simulink model "sm_DynamicCompression"  (R2019b)
settings: Solver=FixedStepDiscrete  StartTime=0.0  StopTime=stop_time  RelTol=1e-3
InitFcn:
  | sm_callback_init
StopFcn:
  | sm_callback_stop
values from neighbouring files (symbols this model uses):
  a = 100*(r^2)    [InitializeCompressionSettings.m]    (also in sm_check_control_signals.m = registers(i).(supplied_fields{j}); sm_check_control_signals_LOCAL_1434.m = registers(i).(supplied_fields{j}))
  B_k_0_init = zeros(1,FIR_0_Uprate)    [sm_callback_init.m]
  B_k_1_init = zeros(1,FIR_0_Uprate)    [sm_callback_init.m]
  B_k_2_init = zeros(1,FIR_0_Uprate)    [sm_callback_init.m]
  B_k_3_init = zeros(1,FIR_0_Uprate)    [sm_callback_init.m]
  B_k_4_init = zeros(1,FIR_0_Uprate)    [sm_callback_init.m]
  B_k_5_init = zeros(1,FIR_0_Uprate)    [sm_callback_init.m]
  calib_bpfs = bpfs    [sm_compression_init.m]
  delayFix = maxDelay-delays    [Initialize_Delay_Values.m]
  F_bits = 28    [TestingLibraryScripts.m]    (also in sm_compression_init.m)
  FIR_0_Size = (ceil(log2(length(calib_bpfs(2:calib_bpfs(1,1)+1 ,1)'))))    [sm_callback_init.m]
  FIR_0_Uprate = 2^FIR_0_Size    [sm_callback_init.m]
  M_bits = 1    [TestingLibraryScripts.m]    (also in sm_compression_init.m = 5)
  M_Bits = M_bits    (= 5)    [sm_compression_init.m]
  mp = sm_init_avalon_signals(mp)    [sm_callback_init.m]
  r_att = nthroot(0.1, s_att)    [sm_compression_init.m]
  r_rel = nthroot(0.1, s_rel)    [sm_compression_init.m]
  recombGain = ones(1,NChans)    [sm_compression_init.m]
  TABLE_SEL_BYPASS_ENABLE = 0    [sm_callback_init.m]
  Ts = mp.Ts    [sm_compression_init.m]
  Ts_system = mp.Ts_system    [sm_compression_init.m]
  W_bits = 32    [TestingLibraryScripts.m]    (also in sm_compression_init.m)
  X_high = 1    [sm_compression_init.m]
undefined symbols (not defined in the file or in its folder): b, c, Gain_Table, ig_eq
libraries: hdlsllib x272, simulink x127, dsphdlfiltering x2
(part 6 of 8)

== system sm_DynamicCompression/dataplane/Avalon Data Processing/Left Channel Processing/recalculate/Nchan_FbankAGC_AID/Compression_4/Compression_Gain_Calc/Linear_Approximation/LSR(N) ==
  NShifts : Inport
  x_in : Inport  Port=2
  Bit Rotate : hdlsllib/Logic and Bit Operations/Bit Rotate  mode=Rotate Right  N=1
      settings: SourceProductName=Simulink  SourceProductBaseCode=SL
  Bit Rotate1 : hdlsllib/Logic and Bit Operations/Bit Rotate  mode=Rotate Right  N=2
      settings: SourceProductName=Simulink  SourceProductBaseCode=SL
  Bit Rotate10 : hdlsllib/Logic and Bit Operations/Bit Rotate  mode=Rotate Right  N=11
      settings: SourceProductName=Simulink  SourceProductBaseCode=SL
  Bit Rotate11 : hdlsllib/Logic and Bit Operations/Bit Rotate  mode=Rotate Right  N=12
      settings: SourceProductName=Simulink  SourceProductBaseCode=SL
  Bit Rotate12 : hdlsllib/Logic and Bit Operations/Bit Rotate  mode=Rotate Right  N=13
      settings: SourceProductName=Simulink  SourceProductBaseCode=SL
  Bit Rotate13 : hdlsllib/Logic and Bit Operations/Bit Rotate  mode=Rotate Right  N=14
      settings: SourceProductName=Simulink  SourceProductBaseCode=SL
  Bit Rotate14 : hdlsllib/Logic and Bit Operations/Bit Rotate  mode=Rotate Right  N=15
      settings: SourceProductName=Simulink  SourceProductBaseCode=SL
  Bit Rotate2 : hdlsllib/Logic and Bit Operations/Bit Rotate  mode=Rotate Right  N=3
      settings: SourceProductName=Simulink  SourceProductBaseCode=SL
  Bit Rotate3 : hdlsllib/Logic and Bit Operations/Bit Rotate  mode=Rotate Right  N=4
      settings: SourceProductName=Simulink  SourceProductBaseCode=SL
  Bit Rotate4 : hdlsllib/Logic and Bit Operations/Bit Rotate  mode=Rotate Right  N=5
      settings: SourceProductName=Simulink  SourceProductBaseCode=SL
  Bit Rotate5 : hdlsllib/Logic and Bit Operations/Bit Rotate  mode=Rotate Right  N=6
      settings: SourceProductName=Simulink  SourceProductBaseCode=SL
  Bit Rotate6 : hdlsllib/Logic and Bit Operations/Bit Rotate  mode=Rotate Right  N=7
      settings: SourceProductName=Simulink  SourceProductBaseCode=SL
  Bit Rotate7 : hdlsllib/Logic and Bit Operations/Bit Rotate  mode=Rotate Right  N=8
      settings: SourceProductName=Simulink  SourceProductBaseCode=SL
  Bit Rotate8 : hdlsllib/Logic and Bit Operations/Bit Rotate  mode=Rotate Right  N=9
      settings: SourceProductName=Simulink  SourceProductBaseCode=SL
  Bit Rotate9 : hdlsllib/Logic and Bit Operations/Bit Rotate  mode=Rotate Right  N=10
      settings: SourceProductName=Simulink  SourceProductBaseCode=SL
  Multiport Switch : MultiPortSwitch  DataPortOrder=Zero-based contiguous  Inputs=16  DiagnosticForDefault=Warning  zeroidx=on
  x_shifted : Outport  VectorParamsAs1DForOutWhenUnconnected=off
  wires:
  NShifts/1 -> Multiport Switch/1
  Multiport Switch/1 -> x_shifted/1
  x_in/1 -> Bit Rotate12/1, Bit Rotate13/1, Bit Rotate14/1, Bit Rotate11/1, Bit Rotate10/1, Bit Rotate9/1, Bit Rotate8/1, Bit Rotate7/1, Bit Rotate5/1, Bit Rotate4/1, Multiport Switch/2, Bit Rotate/1, Bit Rotate1/1, Bit Rotate2/1, Bit Rotate3/1, Bit Rotate6/1
  Bit Rotate/1 -> Multiport Switch/3
  Bit Rotate1/1 -> Multiport Switch/4
  Bit Rotate2/1 -> Multiport Switch/5
  Bit Rotate3/1 -> Multiport Switch/6
  Bit Rotate4/1 -> Multiport Switch/7
  Bit Rotate5/1 -> Multiport Switch/8
  Bit Rotate6/1 -> Multiport Switch/9
  Bit Rotate7/1 -> Multiport Switch/10
  Bit Rotate8/1 -> Multiport Switch/11
  Bit Rotate9/1 -> Multiport Switch/12
  Bit Rotate10/1 -> Multiport Switch/13
  Bit Rotate11/1 -> Multiport Switch/14
  Bit Rotate12/1 -> Multiport Switch/15
  Bit Rotate13/1 -> Multiport Switch/16
  Bit Rotate14/1 -> Multiport Switch/17

== system sm_DynamicCompression/dataplane/Avalon Data Processing/Left Channel Processing/recalculate/Nchan_FbankAGC_AID/Compression_4/Compression_Gain_Calc/LogAddressing/LSL(N) ==
  NShifts : Inport
  x_in : Inport  Port=2
  Bit Rotate : hdlsllib/Logic and Bit Operations/Bit Rotate  mode=Rotate Left  N=1
      settings: SourceProductName=Simulink  SourceProductBaseCode=SL
  Bit Rotate1 : hdlsllib/Logic and Bit Operations/Bit Rotate  mode=Rotate Left  N=2
      settings: SourceProductName=Simulink  SourceProductBaseCode=SL
  Bit Rotate10 : hdlsllib/Logic and Bit Operations/Bit Rotate  mode=Rotate Left  N=11
      settings: SourceProductName=Simulink  SourceProductBaseCode=SL
  Bit Rotate11 : hdlsllib/Logic and Bit Operations/Bit Rotate  mode=Rotate Left  N=12
      settings: SourceProductName=Simulink  SourceProductBaseCode=SL
  Bit Rotate12 : hdlsllib/Logic and Bit Operations/Bit Rotate  mode=Rotate Left  N=13
      settings: SourceProductName=Simulink  SourceProductBaseCode=SL
  Bit Rotate13 : hdlsllib/Logic and Bit Operations/Bit Rotate  mode=Rotate Left  N=14
      settings: SourceProductName=Simulink  SourceProductBaseCode=SL
  Bit Rotate14 : hdlsllib/Logic and Bit Operations/Bit Rotate  mode=Rotate Left  N=15
      settings: SourceProductName=Simulink  SourceProductBaseCode=SL
  Bit Rotate2 : hdlsllib/Logic and Bit Operations/Bit Rotate  mode=Rotate Left  N=3
      settings: SourceProductName=Simulink  SourceProductBaseCode=SL
  Bit Rotate3 : hdlsllib/Logic and Bit Operations/Bit Rotate  mode=Rotate Left  N=4
      settings: SourceProductName=Simulink  SourceProductBaseCode=SL
  Bit Rotate4 : hdlsllib/Logic and Bit Operations/Bit Rotate  mode=Rotate Left  N=5
      settings: SourceProductName=Simulink  SourceProductBaseCode=SL
  Bit Rotate5 : hdlsllib/Logic and Bit Operations/Bit Rotate  mode=Rotate Left  N=6
      settings: SourceProductName=Simulink  SourceProductBaseCode=SL
  Bit Rotate6 : hdlsllib/Logic and Bit Operations/Bit Rotate  mode=Rotate Left  N=7
      settings: SourceProductName=Simulink  SourceProductBaseCode=SL
  Bit Rotate7 : hdlsllib/Logic and Bit Operations/Bit Rotate  mode=Rotate Left  N=8
      settings: SourceProductName=Simulink  SourceProductBaseCode=SL
  Bit Rotate8 : hdlsllib/Logic and Bit Operations/Bit Rotate  mode=Rotate Left  N=9
      settings: SourceProductName=Simulink  SourceProductBaseCode=SL
  Bit Rotate9 : hdlsllib/Logic and Bit Operations/Bit Rotate  mode=Rotate Left  N=10
      settings: SourceProductName=Simulink  SourceProductBaseCode=SL
  Multiport Switch : MultiPortSwitch  DataPortOrder=Zero-based contiguous  Inputs=16  DiagnosticForDefault=Warning  zeroidx=on
  x_shifted : Outport  VectorParamsAs1DForOutWhenUnconnected=off
  wires:
  NShifts/1 -> Multiport Switch/1
  Multiport Switch/1 -> x_shifted/1
  x_in/1 -> Bit Rotate12/1, Bit Rotate13/1, Bit Rotate14/1, Bit Rotate11/1, Bit Rotate10/1, Bit Rotate9/1, Bit Rotate8/1, Bit Rotate7/1, Bit Rotate5/1, Bit Rotate4/1, Multiport Switch/2, Bit Rotate/1, Bit Rotate1/1, Bit Rotate2/1, Bit Rotate3/1, Bit Rotate6/1
  Bit Rotate/1 -> Multiport Switch/3
  Bit Rotate1/1 -> Multiport Switch/4
  Bit Rotate2/1 -> Multiport Switch/5
  Bit Rotate3/1 -> Multiport Switch/6
  Bit Rotate4/1 -> Multiport Switch/7
  Bit Rotate5/1 -> Multiport Switch/8
  Bit Rotate6/1 -> Multiport Switch/9
  Bit Rotate7/1 -> Multiport Switch/10
  Bit Rotate8/1 -> Multiport Switch/11
  Bit Rotate9/1 -> Multiport Switch/12
  Bit Rotate10/1 -> Multiport Switch/13
  Bit Rotate11/1 -> Multiport Switch/14
  Bit Rotate12/1 -> Multiport Switch/15
  Bit Rotate13/1 -> Multiport Switch/16
  Bit Rotate14/1 -> Multiport Switch/17

== system sm_DynamicCompression/dataplane/Avalon Data Processing/Left Channel Processing/recalculate/Nchan_FbankAGC_AID/Compression_5/Compression_Gain_Calc/Linear_Approximation/LSL(N) ==
  NShifts : Inport
  x_in : Inport  Port=2
  Bit Rotate : hdlsllib/Logic and Bit Operations/Bit Rotate  mode=Rotate Left  N=1
      settings: SourceProductName=Simulink  SourceProductBaseCode=SL
  Bit Rotate1 : hdlsllib/Logic and Bit Operations/Bit Rotate  mode=Rotate Left  N=2
      settings: SourceProductName=Simulink  SourceProductBaseCode=SL
  Bit Rotate10 : hdlsllib/Logic and Bit Operations/Bit Rotate  mode=Rotate Left  N=11
      settings: SourceProductName=Simulink  SourceProductBaseCode=SL
  Bit Rotate11 : hdlsllib/Logic and Bit Operations/Bit Rotate  mode=Rotate Left  N=12
      settings: SourceProductName=Simulink  SourceProductBaseCode=SL
  Bit Rotate12 : hdlsllib/Logic and Bit Operations/Bit Rotate  mode=Rotate Left  N=13
      settings: SourceProductName=Simulink  SourceProductBaseCode=SL
  Bit Rotate13 : hdlsllib/Logic and Bit Operations/Bit Rotate  mode=Rotate Left  N=14
      settings: SourceProductName=Simulink  SourceProductBaseCode=SL
  Bit Rotate14 : hdlsllib/Logic and Bit Operations/Bit Rotate  mode=Rotate Left  N=15
      settings: SourceProductName=Simulink  SourceProductBaseCode=SL
  Bit Rotate2 : hdlsllib/Logic and Bit Operations/Bit Rotate  mode=Rotate Left  N=3
      settings: SourceProductName=Simulink  SourceProductBaseCode=SL
  Bit Rotate3 : hdlsllib/Logic and Bit Operations/Bit Rotate  mode=Rotate Left  N=4
      settings: SourceProductName=Simulink  SourceProductBaseCode=SL
  Bit Rotate4 : hdlsllib/Logic and Bit Operations/Bit Rotate  mode=Rotate Left  N=5
      settings: SourceProductName=Simulink  SourceProductBaseCode=SL
  Bit Rotate5 : hdlsllib/Logic and Bit Operations/Bit Rotate  mode=Rotate Left  N=6
      settings: SourceProductName=Simulink  SourceProductBaseCode=SL
  Bit Rotate6 : hdlsllib/Logic and Bit Operations/Bit Rotate  mode=Rotate Left  N=7
      settings: SourceProductName=Simulink  SourceProductBaseCode=SL
  Bit Rotate7 : hdlsllib/Logic and Bit Operations/Bit Rotate  mode=Rotate Left  N=8
      settings: SourceProductName=Simulink  SourceProductBaseCode=SL
  Bit Rotate8 : hdlsllib/Logic and Bit Operations/Bit Rotate  mode=Rotate Left  N=9
      settings: SourceProductName=Simulink  SourceProductBaseCode=SL
  Bit Rotate9 : hdlsllib/Logic and Bit Operations/Bit Rotate  mode=Rotate Left  N=10
      settings: SourceProductName=Simulink  SourceProductBaseCode=SL
  Multiport Switch : MultiPortSwitch  DataPortOrder=Zero-based contiguous  Inputs=16  DiagnosticForDefault=Warning  zeroidx=on
  x_shifted : Outport  VectorParamsAs1DForOutWhenUnconnected=off
  wires:
  NShifts/1 -> Multiport Switch/1
  Multiport Switch/1 -> x_shifted/1
  x_in/1 -> Bit Rotate12/1, Bit Rotate13/1, Bit Rotate14/1, Bit Rotate11/1, Bit Rotate10/1, Bit Rotate9/1, Bit Rotate8/1, Bit Rotate7/1, Bit Rotate5/1, Bit Rotate4/1, Multiport Switch/2, Bit Rotate/1, Bit Rotate1/1, Bit Rotate2/1, Bit Rotate3/1, Bit Rotate6/1
  Bit Rotate/1 -> Multiport Switch/3
  Bit Rotate1/1 -> Multiport Switch/4
  Bit Rotate2/1 -> Multiport Switch/5
  Bit Rotate3/1 -> Multiport Switch/6
  Bit Rotate4/1 -> Multiport Switch/7
  Bit Rotate5/1 -> Multiport Switch/8
  Bit Rotate6/1 -> Multiport Switch/9
  Bit Rotate7/1 -> Multiport Switch/10
  Bit Rotate8/1 -> Multiport Switch/11
  Bit Rotate9/1 -> Multiport Switch/12
  Bit Rotate10/1 -> Multiport Switch/13
  Bit Rotate11/1 -> Multiport Switch/14
  Bit Rotate12/1 -> Multiport Switch/15
  Bit Rotate13/1 -> Multiport Switch/16
  Bit Rotate14/1 -> Multiport Switch/17

== system sm_DynamicCompression/dataplane/Avalon Data Processing/Left Channel Processing/recalculate/Nchan_FbankAGC_AID/Compression_5/Compression_Gain_Calc/Linear_Approximation/LSR(N) ==
  NShifts : Inport
  x_in : Inport  Port=2
  Bit Rotate : hdlsllib/Logic and Bit Operations/Bit Rotate  mode=Rotate Right  N=1
      settings: SourceProductName=Simulink  SourceProductBaseCode=SL
  Bit Rotate1 : hdlsllib/Logic and Bit Operations/Bit Rotate  mode=Rotate Right  N=2
      settings: SourceProductName=Simulink  SourceProductBaseCode=SL
  Bit Rotate10 : hdlsllib/Logic and Bit Operations/Bit Rotate  mode=Rotate Right  N=11
      settings: SourceProductName=Simulink  SourceProductBaseCode=SL
  Bit Rotate11 : hdlsllib/Logic and Bit Operations/Bit Rotate  mode=Rotate Right  N=12
      settings: SourceProductName=Simulink  SourceProductBaseCode=SL
  Bit Rotate12 : hdlsllib/Logic and Bit Operations/Bit Rotate  mode=Rotate Right  N=13
      settings: SourceProductName=Simulink  SourceProductBaseCode=SL
  Bit Rotate13 : hdlsllib/Logic and Bit Operations/Bit Rotate  mode=Rotate Right  N=14
      settings: SourceProductName=Simulink  SourceProductBaseCode=SL
  Bit Rotate14 : hdlsllib/Logic and Bit Operations/Bit Rotate  mode=Rotate Right  N=15
      settings: SourceProductName=Simulink  SourceProductBaseCode=SL
  Bit Rotate2 : hdlsllib/Logic and Bit Operations/Bit Rotate  mode=Rotate Right  N=3
      settings: SourceProductName=Simulink  SourceProductBaseCode=SL
  Bit Rotate3 : hdlsllib/Logic and Bit Operations/Bit Rotate  mode=Rotate Right  N=4
      settings: SourceProductName=Simulink  SourceProductBaseCode=SL
  Bit Rotate4 : hdlsllib/Logic and Bit Operations/Bit Rotate  mode=Rotate Right  N=5
      settings: SourceProductName=Simulink  SourceProductBaseCode=SL
  Bit Rotate5 : hdlsllib/Logic and Bit Operations/Bit Rotate  mode=Rotate Right  N=6
      settings: SourceProductName=Simulink  SourceProductBaseCode=SL
  Bit Rotate6 : hdlsllib/Logic and Bit Operations/Bit Rotate  mode=Rotate Right  N=7
      settings: SourceProductName=Simulink  SourceProductBaseCode=SL
  Bit Rotate7 : hdlsllib/Logic and Bit Operations/Bit Rotate  mode=Rotate Right  N=8
      settings: SourceProductName=Simulink  SourceProductBaseCode=SL
  Bit Rotate8 : hdlsllib/Logic and Bit Operations/Bit Rotate  mode=Rotate Right  N=9
      settings: SourceProductName=Simulink  SourceProductBaseCode=SL
  Bit Rotate9 : hdlsllib/Logic and Bit Operations/Bit Rotate  mode=Rotate Right  N=10
      settings: SourceProductName=Simulink  SourceProductBaseCode=SL
  Multiport Switch : MultiPortSwitch  DataPortOrder=Zero-based contiguous  Inputs=16  DiagnosticForDefault=Warning  zeroidx=on
  x_shifted : Outport  VectorParamsAs1DForOutWhenUnconnected=off
  wires:
  NShifts/1 -> Multiport Switch/1
  Multiport Switch/1 -> x_shifted/1
  x_in/1 -> Bit Rotate12/1, Bit Rotate13/1, Bit Rotate14/1, Bit Rotate11/1, Bit Rotate10/1, Bit Rotate9/1, Bit Rotate8/1, Bit Rotate7/1, Bit Rotate5/1, Bit Rotate4/1, Multiport Switch/2, Bit Rotate/1, Bit Rotate1/1, Bit Rotate2/1, Bit Rotate3/1, Bit Rotate6/1
  Bit Rotate/1 -> Multiport Switch/3
  Bit Rotate1/1 -> Multiport Switch/4
  Bit Rotate2/1 -> Multiport Switch/5
  Bit Rotate3/1 -> Multiport Switch/6
  Bit Rotate4/1 -> Multiport Switch/7
  Bit Rotate5/1 -> Multiport Switch/8
  Bit Rotate6/1 -> Multiport Switch/9
  Bit Rotate7/1 -> Multiport Switch/10
  Bit Rotate8/1 -> Multiport Switch/11
  Bit Rotate9/1 -> Multiport Switch/12
  Bit Rotate10/1 -> Multiport Switch/13
  Bit Rotate11/1 -> Multiport Switch/14
  Bit Rotate12/1 -> Multiport Switch/15
  Bit Rotate13/1 -> Multiport Switch/16
  Bit Rotate14/1 -> Multiport Switch/17

== system sm_DynamicCompression/dataplane/Avalon Data Processing/Left Channel Processing/recalculate/Nchan_FbankAGC_AID/Compression_5/Compression_Gain_Calc/LogAddressing/LSL(N) ==
  NShifts : Inport
  x_in : Inport  Port=2
  Bit Rotate : hdlsllib/Logic and Bit Operations/Bit Rotate  mode=Rotate Left  N=1
      settings: SourceProductName=Simulink  SourceProductBaseCode=SL
  Bit Rotate1 : hdlsllib/Logic and Bit Operations/Bit Rotate  mode=Rotate Left  N=2
      settings: SourceProductName=Simulink  SourceProductBaseCode=SL
  Bit Rotate10 : hdlsllib/Logic and Bit Operations/Bit Rotate  mode=Rotate Left  N=11
      settings: SourceProductName=Simulink  SourceProductBaseCode=SL
  Bit Rotate11 : hdlsllib/Logic and Bit Operations/Bit Rotate  mode=Rotate Left  N=12
      settings: SourceProductName=Simulink  SourceProductBaseCode=SL
  Bit Rotate12 : hdlsllib/Logic and Bit Operations/Bit Rotate  mode=Rotate Left  N=13
      settings: SourceProductName=Simulink  SourceProductBaseCode=SL
  Bit Rotate13 : hdlsllib/Logic and Bit Operations/Bit Rotate  mode=Rotate Left  N=14
      settings: SourceProductName=Simulink  SourceProductBaseCode=SL
  Bit Rotate14 : hdlsllib/Logic and Bit Operations/Bit Rotate  mode=Rotate Left  N=15
      settings: SourceProductName=Simulink  SourceProductBaseCode=SL
  Bit Rotate2 : hdlsllib/Logic and Bit Operations/Bit Rotate  mode=Rotate Left  N=3
      settings: SourceProductName=Simulink  SourceProductBaseCode=SL
  Bit Rotate3 : hdlsllib/Logic and Bit Operations/Bit Rotate  mode=Rotate Left  N=4
      settings: SourceProductName=Simulink  SourceProductBaseCode=SL
  Bit Rotate4 : hdlsllib/Logic and Bit Operations/Bit Rotate  mode=Rotate Left  N=5
      settings: SourceProductName=Simulink  SourceProductBaseCode=SL
  Bit Rotate5 : hdlsllib/Logic and Bit Operations/Bit Rotate  mode=Rotate Left  N=6
      settings: SourceProductName=Simulink  SourceProductBaseCode=SL
  Bit Rotate6 : hdlsllib/Logic and Bit Operations/Bit Rotate  mode=Rotate Left  N=7
      settings: SourceProductName=Simulink  SourceProductBaseCode=SL
  Bit Rotate7 : hdlsllib/Logic and Bit Operations/Bit Rotate  mode=Rotate Left  N=8
      settings: SourceProductName=Simulink  SourceProductBaseCode=SL
  Bit Rotate8 : hdlsllib/Logic and Bit Operations/Bit Rotate  mode=Rotate Left  N=9
      settings: SourceProductName=Simulink  SourceProductBaseCode=SL
  Bit Rotate9 : hdlsllib/Logic and Bit Operations/Bit Rotate  mode=Rotate Left  N=10
      settings: SourceProductName=Simulink  SourceProductBaseCode=SL
  Multiport Switch : MultiPortSwitch  DataPortOrder=Zero-based contiguous  Inputs=16  DiagnosticForDefault=Warning  zeroidx=on
  x_shifted : Outport  VectorParamsAs1DForOutWhenUnconnected=off
  wires:
  NShifts/1 -> Multiport Switch/1
  Multiport Switch/1 -> x_shifted/1
  x_in/1 -> Bit Rotate12/1, Bit Rotate13/1, Bit Rotate14/1, Bit Rotate11/1, Bit Rotate10/1, Bit Rotate9/1, Bit Rotate8/1, Bit Rotate7/1, Bit Rotate5/1, Bit Rotate4/1, Multiport Switch/2, Bit Rotate/1, Bit Rotate1/1, Bit Rotate2/1, Bit Rotate3/1, Bit Rotate6/1
  Bit Rotate/1 -> Multiport Switch/3
  Bit Rotate1/1 -> Multiport Switch/4
  Bit Rotate2/1 -> Multiport Switch/5
  Bit Rotate3/1 -> Multiport Switch/6
  Bit Rotate4/1 -> Multiport Switch/7
  Bit Rotate5/1 -> Multiport Switch/8
  Bit Rotate6/1 -> Multiport Switch/9
  Bit Rotate7/1 -> Multiport Switch/10
  Bit Rotate8/1 -> Multiport Switch/11
  Bit Rotate9/1 -> Multiport Switch/12
  Bit Rotate10/1 -> Multiport Switch/13
  Bit Rotate11/1 -> Multiport Switch/14
  Bit Rotate12/1 -> Multiport Switch/15
  Bit Rotate13/1 -> Multiport Switch/16
  Bit Rotate14/1 -> Multiport Switch/17

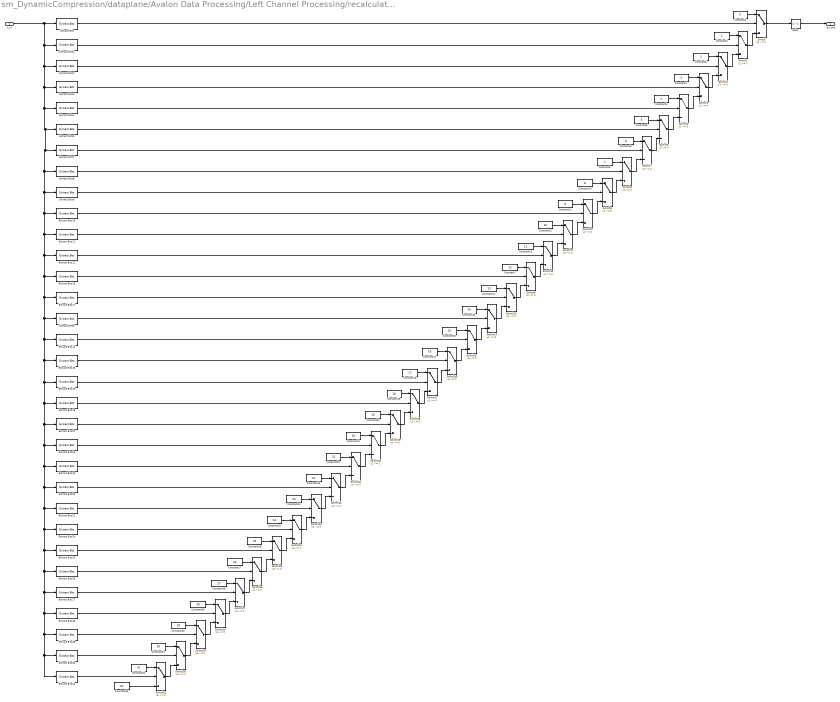
== system sm_DynamicCompression/dataplane/Avalon Data Processing/Left Channel Processing/recalculate/Nchan_FbankAGC_AID/Compression_1/Compression_Gain_Calc/LogAddressing/fxpt_lzc_W32/LZC32 ==
  x_in : Inport
  Constant1 : Constant  OutDataTypeStr=fixdt(0,6,0)  SampleTime=Ts_system
  Constant10 : Constant  Value=8  OutDataTypeStr=fixdt(0,6,0)  SampleTime=Ts_system
  Constant11 : Constant  Value=9  OutDataTypeStr=fixdt(0,6,0)  SampleTime=Ts_system
  Constant12 : Constant  Value=10  OutDataTypeStr=fixdt(0,6,0)  SampleTime=Ts_system
  Constant13 : Constant  Value=11  OutDataTypeStr=fixdt(0,6,0)  SampleTime=Ts_system
  Constant14 : Constant  Value=13  OutDataTypeStr=fixdt(0,6,0)  SampleTime=Ts_system
  Constant15 : Constant  Value=14  OutDataTypeStr=fixdt(0,6,0)  SampleTime=Ts_system
  Constant16 : Constant  Value=15  OutDataTypeStr=fixdt(0,6,0)  SampleTime=Ts_system
  Constant17 : Constant  Value=16  OutDataTypeStr=fixdt(0,6,0)  SampleTime=Ts_system
  Constant18 : Constant  Value=17  OutDataTypeStr=fixdt(0,6,0)  SampleTime=Ts_system
  Constant19 : Constant  Value=18  OutDataTypeStr=fixdt(0,6,0)  SampleTime=Ts_system
  Constant2 : Constant  Value=0  OutDataTypeStr=fixdt(0,6,0)  SampleTime=Ts_system
  Constant20 : Constant  Value=19  OutDataTypeStr=fixdt(0,6,0)  SampleTime=Ts_system
  Constant21 : Constant  Value=20  OutDataTypeStr=fixdt(0,6,0)  SampleTime=Ts_system
  Constant22 : Constant  Value=21  OutDataTypeStr=fixdt(0,6,0)  SampleTime=Ts_system
  Constant23 : Constant  Value=22  OutDataTypeStr=fixdt(0,6,0)  SampleTime=Ts_system
  Constant24 : Constant  Value=23  OutDataTypeStr=fixdt(0,6,0)  SampleTime=Ts_system
  Constant25 : Constant  Value=24  OutDataTypeStr=fixdt(0,6,0)  SampleTime=Ts_system
  Constant26 : Constant  Value=25  OutDataTypeStr=fixdt(0,6,0)  SampleTime=Ts_system
  Constant27 : Constant  Value=26  OutDataTypeStr=fixdt(0,6,0)  SampleTime=Ts_system
  Constant28 : Constant  Value=27  OutDataTypeStr=fixdt(0,6,0)  SampleTime=Ts_system
  Constant29 : Constant  Value=28  OutDataTypeStr=fixdt(0,6,0)  SampleTime=Ts_system
  Constant3 : Constant  Value=2  OutDataTypeStr=fixdt(0,6,0)  SampleTime=Ts_system
  Constant30 : Constant  Value=29  OutDataTypeStr=fixdt(0,6,0)  SampleTime=Ts_system
  Constant31 : Constant  Value=30  OutDataTypeStr=fixdt(0,6,0)  SampleTime=Ts_system
  Constant32 : Constant  Value=31  OutDataTypeStr=fixdt(0,6,0)  SampleTime=Ts_system
  Constant33 : Constant  Value=32  OutDataTypeStr=fixdt(0,6,0)  SampleTime=Ts_system
  Constant4 : Constant  Value=3  OutDataTypeStr=fixdt(0,6,0)  SampleTime=Ts_system
  Constant5 : Constant  Value=4  OutDataTypeStr=fixdt(0,6,0)  SampleTime=Ts_system
  Constant6 : Constant  Value=5  OutDataTypeStr=fixdt(0,6,0)  SampleTime=Ts_system
  Constant7 : Constant  Value=12  OutDataTypeStr=fixdt(0,6,0)  SampleTime=Ts_system
  Constant8 : Constant  Value=6  OutDataTypeStr=fixdt(0,6,0)  SampleTime=Ts_system
  Constant9 : Constant  Value=7  OutDataTypeStr=fixdt(0,6,0)  SampleTime=Ts_system
  Delay : Delay  DelayLength=1  InitialCondition=3
  Extract Bits : simulink/Logic and Bit Operations/Extract Bits  bitsToExtract=Range of bits  numBits=8  bitIdxRange=[31 31]  outScalingMode=Treat bit field as an integer
      settings: SourceProductName=Simulink
  Extract Bits1 : simulink/Logic and Bit Operations/Extract Bits  bitsToExtract=Range of bits  numBits=8  bitIdxRange=[30 30]  outScalingMode=Treat bit field as an integer
      settings: SourceProductName=Simulink
  Extract Bits10 : simulink/Logic and Bit Operations/Extract Bits  bitsToExtract=Range of bits  numBits=8  bitIdxRange=[22 22]  outScalingMode=Treat bit field as an integer
      settings: SourceProductName=Simulink
  Extract Bits11 : simulink/Logic and Bit Operations/Extract Bits  bitsToExtract=Range of bits  numBits=8  bitIdxRange=[21 21]  outScalingMode=Treat bit field as an integer
      settings: SourceProductName=Simulink
  Extract Bits12 : simulink/Logic and Bit Operations/Extract Bits  bitsToExtract=Range of bits  numBits=8  bitIdxRange=[20 20]  outScalingMode=Treat bit field as an integer
      settings: SourceProductName=Simulink
  Extract Bits13 : simulink/Logic and Bit Operations/Extract Bits  bitsToExtract=Range of bits  numBits=8  bitIdxRange=[19 19]  outScalingMode=Treat bit field as an integer
      settings: SourceProductName=Simulink
  Extract Bits14 : simulink/Logic and Bit Operations/Extract Bits  bitsToExtract=Range of bits  numBits=8  bitIdxRange=[16 16]  outScalingMode=Treat bit field as an integer
      settings: SourceProductName=Simulink
  Extract Bits15 : simulink/Logic and Bit Operations/Extract Bits  bitsToExtract=Range of bits  numBits=8  bitIdxRange=[15 15]  outScalingMode=Treat bit field as an integer
      settings: SourceProductName=Simulink
  Extract Bits16 : simulink/Logic and Bit Operations/Extract Bits  bitsToExtract=Range of bits  numBits=8  bitIdxRange=[14 14]  outScalingMode=Treat bit field as an integer
      settings: SourceProductName=Simulink
  Extract Bits17 : simulink/Logic and Bit Operations/Extract Bits  bitsToExtract=Range of bits  numBits=8  bitIdxRange=[18 18]  outScalingMode=Treat bit field as an integer
      settings: SourceProductName=Simulink
  Extract Bits18 : simulink/Logic and Bit Operations/Extract Bits  bitsToExtract=Range of bits  numBits=8  bitIdxRange=[13 13]  outScalingMode=Treat bit field as an integer
      settings: SourceProductName=Simulink
  Extract Bits19 : simulink/Logic and Bit Operations/Extract Bits  bitsToExtract=Range of bits  numBits=8  bitIdxRange=[10 10]  outScalingMode=Treat bit field as an integer
      settings: SourceProductName=Simulink
  Extract Bits2 : simulink/Logic and Bit Operations/Extract Bits  bitsToExtract=Range of bits  numBits=8  bitIdxRange=[29 29]  outScalingMode=Treat bit field as an integer
      settings: SourceProductName=Simulink
  Extract Bits20 : simulink/Logic and Bit Operations/Extract Bits  bitsToExtract=Range of bits  numBits=8  bitIdxRange=[9 9]  outScalingMode=Treat bit field as an integer
      settings: SourceProductName=Simulink
  Extract Bits21 : simulink/Logic and Bit Operations/Extract Bits  bitsToExtract=Range of bits  numBits=8  bitIdxRange=[8 8]  outScalingMode=Treat bit field as an integer
      settings: SourceProductName=Simulink
  Extract Bits22 : simulink/Logic and Bit Operations/Extract Bits  bitsToExtract=Range of bits  numBits=8  bitIdxRange=[12 12]  outScalingMode=Treat bit field as an integer
      settings: SourceProductName=Simulink
  Extract Bits23 : simulink/Logic and Bit Operations/Extract Bits  bitsToExtract=Range of bits  numBits=8  bitIdxRange=[11 11]  outScalingMode=Treat bit field as an integer
      settings: SourceProductName=Simulink
  Extract Bits24 : simulink/Logic and Bit Operations/Extract Bits  bitsToExtract=Range of bits  numBits=8  bitIdxRange=[7 7]  outScalingMode=Treat bit field as an integer
      settings: SourceProductName=Simulink
  Extract Bits25 : simulink/Logic and Bit Operations/Extract Bits  bitsToExtract=Range of bits  numBits=8  bitIdxRange=[6 6]  outScalingMode=Treat bit field as an integer
      settings: SourceProductName=Simulink
  Extract Bits26 : simulink/Logic and Bit Operations/Extract Bits  bitsToExtract=Range of bits  numBits=8  bitIdxRange=[5 5]  outScalingMode=Treat bit field as an integer
      settings: SourceProductName=Simulink
  Extract Bits27 : simulink/Logic and Bit Operations/Extract Bits  bitsToExtract=Range of bits  numBits=8  bitIdxRange=[4 4]  outScalingMode=Treat bit field as an integer
      settings: SourceProductName=Simulink
  Extract Bits28 : simulink/Logic and Bit Operations/Extract Bits  bitsToExtract=Range of bits  numBits=8  bitIdxRange=[3 3]  outScalingMode=Treat bit field as an integer
      settings: SourceProductName=Simulink
  Extract Bits29 : simulink/Logic and Bit Operations/Extract Bits  bitsToExtract=Range of bits  numBits=8  bitIdxRange=[2 2]  outScalingMode=Treat bit field as an integer
      settings: SourceProductName=Simulink
  Extract Bits3 : simulink/Logic and Bit Operations/Extract Bits  bitsToExtract=Range of bits  numBits=8  bitIdxRange=[28 28]  outScalingMode=Treat bit field as an integer
      settings: SourceProductName=Simulink
  Extract Bits30 : simulink/Logic and Bit Operations/Extract Bits  bitsToExtract=Range of bits  numBits=8  bitIdxRange=[1 1]  outScalingMode=Treat bit field as an integer
      settings: SourceProductName=Simulink
  Extract Bits31 : simulink/Logic and Bit Operations/Extract Bits  bitsToExtract=Range of bits  numBits=8  bitIdxRange=[0 0]  outScalingMode=Treat bit field as an integer
      settings: SourceProductName=Simulink
  Extract Bits4 : simulink/Logic and Bit Operations/Extract Bits  bitsToExtract=Range of bits  numBits=8  bitIdxRange=[27 27]  outScalingMode=Treat bit field as an integer
      settings: SourceProductName=Simulink
  Extract Bits5 : simulink/Logic and Bit Operations/Extract Bits  bitsToExtract=Range of bits  numBits=8  bitIdxRange=[26 26]  outScalingMode=Treat bit field as an integer
      settings: SourceProductName=Simulink
  Extract Bits6 : simulink/Logic and Bit Operations/Extract Bits  bitsToExtract=Range of bits  numBits=8  bitIdxRange=[17 17]  outScalingMode=Treat bit field as an integer
      settings: SourceProductName=Simulink
  Extract Bits7 : simulink/Logic and Bit Operations/Extract Bits  bitsToExtract=Range of bits  numBits=8  bitIdxRange=[25 25]  outScalingMode=Treat bit field as an integer
      settings: SourceProductName=Simulink
  Extract Bits8 : simulink/Logic and Bit Operations/Extract Bits  bitsToExtract=Range of bits  numBits=8  bitIdxRange=[24 24]  outScalingMode=Treat bit field as an integer
      settings: SourceProductName=Simulink
  Extract Bits9 : simulink/Logic and Bit Operations/Extract Bits  bitsToExtract=Range of bits  numBits=8  bitIdxRange=[23 23]  outScalingMode=Treat bit field as an integer
      settings: SourceProductName=Simulink
  Switch{,1..31} (32 alike) : Switch  Criteria=u2 ~= 0
  lzc_out : Outport  VectorParamsAs1DForOutWhenUnconnected=off
  wires:
  Delay/1 -> lzc_out/1
  Switch/1 -> Delay/1
  Extract Bits3/1 -> Switch3/2
  Constant6/1 -> Switch5/1
  Constant5/1 -> Switch4/1
  Switch1/1 -> Switch/3
  Extract Bits16/1 -> Switch17/2
  Constant19/1 -> Switch18/1
  Constant21/1 -> Switch20/1
  Constant20/1 -> Switch19/1
  Switch23/1 -> Switch22/3
  Switch22/1 -> Switch21/3
  Constant24/1 -> Switch23/1
  Constant23/1 -> Switch22/1
  Constant9/1 -> Switch8/1
  Constant13/1 -> Switch12/1
  Switch10/1 -> Switch9/3
  Switch21/1 -> Switch20/3
  Constant12/1 -> Switch11/1
  Switch8/1 -> Switch7/3
  Switch12/1 -> Switch11/3
  Constant10/1 -> Switch9/1
  Constant25/1 -> Switch24/1
  Switch25/1 -> Switch24/3
  Constant27/1 -> Switch26/1
  Constant26/1 -> Switch25/1
  Constant32/1 -> Switch31/1
  Switch27/1 -> Switch26/3
  Constant29/1 -> Switch28/1
  Constant30/1 -> Switch29/1
  Constant7/1 -> Switch6/1
  Switch17/1 -> Switch16/3
  Switch13/1 -> Switch6/3
  Switch30/1 -> Switch29/3
  Switch15/1 -> Switch14/3
  Constant22/1 -> Switch21/1
  Constant2/1 -> Switch/1
  Extract Bits7/1 -> Switch7/2
  Extract Bits8/1 -> Switch8/2
  Extract Bits10/1 -> Switch10/2
  Constant4/1 -> Switch3/1
  Constant18/1 -> Switch17/1
  Extract Bits11/1 -> Switch11/2
  Extract Bits13/1 -> Switch6/2
  Switch7/1 -> Switch5/3
  Extract Bits9/1 -> Switch9/2
  Switch19/1 -> Switch18/3
  Switch31/1 -> Switch30/3
  Switch9/1 -> Switch8/3
  Extract Bits29/1 -> Switch29/2
  Switch16/1 -> Switch15/3
  Extract Bits25/1 -> Switch25/2
  Constant8/1 -> Switch7/1
  Constant11/1 -> Switch10/1
  Switch28/1 -> Switch27/3
  Extract Bits24/1 -> Switch24/2
  Extract Bits17/1 -> Switch13/2
  Extract Bits12/1 -> Switch12/2
  Switch11/1 -> Switch10/3
  Extract Bits22/1 -> Switch19/2
  Extract Bits26/1 -> Switch26/2
  Extract Bits20/1 -> Switch22/2
  Extract Bits18/1 -> Switch18/2
  Extract Bits5/1 -> Switch5/2
  Constant17/1 -> Switch16/1
  Extract Bits6/1 -> Switch14/2
  Constant15/1 -> Switch14/1
  Extract Bits23/1 -> Switch20/2
  Extract Bits14/1 -> Switch15/2
  Switch20/1 -> Switch19/3
  Switch29/1 -> Switch28/3
  Extract Bits28/1 -> Switch28/2
  Extract Bits21/1 -> Switch23/2
  Switch18/1 -> Switch17/3
  Switch26/1 -> Switch25/3
  Extract Bits2/1 -> Switch2/2
  Extract Bits19/1 -> Switch21/2
  Switch3/1 -> Switch2/3
  Extract Bits15/1 -> Switch16/2
  Constant1/1 -> Switch1/1
  Extract Bits30/1 -> Switch30/2
  Constant3/1 -> Switch2/1
  Extract Bits4/1 -> Switch4/2
  Constant16/1 -> Switch15/1
  Extract Bits27/1 -> Switch27/2
  Switch14/1 -> Switch13/3
  Switch24/1 -> Switch23/3
  Constant33/1 -> Switch31/3
  Extract Bits/1 -> Switch/2
  Constant31/1 -> Switch30/1
  Constant14/1 -> Switch13/1
  Switch5/1 -> Switch4/3
  Switch6/1 -> Switch12/3
  Extract Bits1/1 -> Switch1/2
  Switch2/1 -> Switch1/3
  Constant28/1 -> Switch27/1
  Extract Bits31/1 -> Switch31/2
  Switch4/1 -> Switch3/3
  x_in/1 -> Extract Bits/1, Extract Bits1/1, Extract Bits2/1, Extract Bits3/1, Extract Bits4/1, Extract Bits5/1, Extract Bits7/1, Extract Bits8/1, Extract Bits9/1, Extract Bits10/1, Extract Bits11/1, Extract Bits12/1, Extract Bits13/1, Extract Bits17/1, Extract Bits6/1, Extract Bits14/1, Extract Bits15/1, Extract Bits16/1, Extract Bits18/1, Extract Bits22/1, Extract Bits23/1, Extract Bits19/1, Extract Bits20/1, Extract Bits21/1, Extract Bits24/1, Extract Bits25/1, Extract Bits26/1, Extract Bits27/1, Extract Bits28/1, Extract Bits29/1, Extract Bits30/1, Extract Bits31/1

== matlab function sm_DynamicCompression/dataplane/Avalon Data Processing/Left Channel Processing/recalculate/Nchan_FbankAGC_AID/Compression_2/Compression_Gain_Calc/LogAddressing/MATLAB Function ==
  data: x input; lzc_count output
function lzc_count = fcn(x)
%#codegen

% -- Binary Bisection Tree (Divide & Conquer)
if bitorreduce(x, 40, 21) == 1 %       if ((b39 or b38 or b37 or b36 or b35 or b34 or b33 or b32 or b31 or b30 or b29 or b28 or b27 or b26 or b25 or b24 or b23 or b22 or b21 or b20) = '1') then   -- check bit range [39  20]
    if bitorreduce(x, 40, 31) == 1%             if ((b39 or b38 or b37 or b36 or b35 or b34 or b33 or b32 or b31 or b30) = '1') then   -- check bit range [39  30]
        if bitorreduce(x, 40, 36) == 1%                 if ((b39 or b38 or b37 or b36 or b35) = '1') then   -- check bit range [39  35]
            if bitorreduce(x, 40, 38) == 1%                     if ((b39 or b38 or b37) = '1') then   -- check bit range [39  37]
                if bitorreduce(x, 40, 39) == 1%                         if ((b39 or b38) = '1') then   -- check bit range [39  38]
                    if bitorreduce(x, 40, 40) == 1%                             if (b39 = '1') then   -- [39]
                        lzc_count = fi(0,0,6,0);%                                 lzc_count <= "000000";  -- lzc = 0
                    else%                             else  -- check bit range [38]
                        lzc_count = fi(1,0,6,0);%                                 lzc_count <= "000001";  -- lzc = 1
                    end%                             end if;
                else%                         else  -- check bit range [37]
                    lzc_count = fi(2,0,6,0);%                             lzc_count <= "000010";  -- lzc = 2
                end%                         end if;
            else%                     else  -- check bit range [36  35]
                if bitorreduce(x, 37, 37) == 1%                         if (b36 = '1') then   -- [36]
                    lzc_count = fi(3,0,6,0);%                             lzc_count <= "000011";  -- lzc = 3
                else%                         else  -- check bit range [35]
                    lzc_count = fi(4,0,6,0);%                             lzc_count <= "000100";  -- lzc = 4
                end%                         end if;
            end%                     end if;
        else%                 else  -- check bit range [34  30]
            if bitorreduce(x, 35, 33) == 1%                     if ((b34 or b33 or b32) = '1') then   -- check bit range [34  32]
                if bitorreduce(x, 35, 34) == 1%                         if ((b34 or b33) = '1') then   -- check bit range [34  33]
                    if bitorreduce(x, 35, 35) == 1%                             if (b34 = '1') then   -- [34]
                        lzc_count = fi(5,0,6,0);%                                 lzc_count <= "000101";  -- lzc = 5
                    else%                             else  -- check bit range [33]
                        lzc_count = fi(6,0,6,0);%                                 lzc_count <= "000110";  -- lzc = 6
                    end%                             end if;
                else%                         else  -- check bit range [32]
                    lzc_count = fi(7,0,6,0);%                             lzc_count <= "000111";  -- lzc = 7
                end%                         end if;
            else%                     else  -- check bit range [31  30]
                if bitorreduce(x, 32, 32) == 1%                         if (b31 = '1') then   -- [31]
                    lzc_count = fi(8,0,6,0);%                             lzc_count <= "001000";  -- lzc = 8
                else%                         else  -- check bit range [30]
                    lzc_count = fi(9,0,6,0);%                             lzc_count <= "001001";  -- lzc = 9
                end%                         end if;
            end%                     end if;
        end%                 end if;
    else%             else  -- check bit range [29  20]
        if bitorreduce(x, 30, 26) == 1%                 if ((b29 or b28 or b27 or b26 or b25) = '1') then   -- check bit range [29  25]
            if bitorreduce(x, 30, 28) == 1%                     if ((b29 or b28 or b27) = '1') then   -- check bit range [29  27]
                if bitorreduce(x, 30, 29) == 1%                         if ((b29 or b28) = '1') then   -- check bit range [29  28]
                    if bitorreduce(x, 30, 30) == 1%                             if (b29 = '1') then   -- [29]
                        lzc_count = fi(10,0,6,0);%                                 lzc_count <= "001010";  -- lzc = 10
                    else%                             else  -- check bit range [28]
                        lzc_count = fi(11,0,6,0);%                                 lzc_count <= "001011";  -- lzc = 11
                    end%                             end if;
                else%                         else  -- check bit range [27]
                    lzc_count = fi(12,0,6,0);%                             lzc_count <= "001100";  -- lzc = 12
                end%                         end if;
            else%                     else  -- check bit range [26  25]
                if bitorreduce(x, 27, 27) == 1%                         if (b26 = '1') then   -- [26]
                    lzc_count = fi(13,0,6,0);%                             lzc_count <= "001101";  -- lzc = 13
                else%                         else  -- check bit range [25]
                    lzc_count = fi(14,0,6,0);%                             lzc_count <= "001110";  -- lzc = 14
                end%                         end if;
            end%                     end if;
        else%                 else  -- check bit range [24  20]
            if bitorreduce(x, 25, 23) == 1%                     if ((b24 or b23 or b22) = '1') then   -- check bit range [24  22]
                if bitorreduce(x, 25, 24) == 1%                         if ((b24 or b23) = '1') then   -- check bit range [24  23]
                    if bitorreduce(x, 25, 25) == 1%                             if (b24 = '1') then   -- [24]
                        lzc_count = fi(15,0,6,0);%                                 lzc_count <= "001111";  -- lzc = 15
                    else%                             else  -- check bit range [23]
                        lzc_count = fi(16,0,6,0);%                                 lzc_count <= "010000";  -- lzc = 16
                    end%                             end if;
                else%                         else  -- check bit range [22]
                    lzc_count = fi(17,0,6,0);%                             lzc_count <= "010001";  -- lzc = 17
                end%                         end if;
            else%                     else  -- check bit range [21  20]
                if bitorreduce(x, 22, 22) == 1%                         if (b21 = '1') then   -- [21]
                    lzc_count = fi(18,0,6,0);%                             lzc_count <= "010010";  -- lzc = 18
                else%                         else  -- check bit range [20]
                    lzc_count = fi(19,0,6,0);%                             lzc_count <= "010011";  -- lzc = 19
                end%                         end if;
            end%                     end if;
        end%                 end if;
    end%             end if;
else%         else  -- check bit range [19   0]
    if bitorreduce(x, 20, 11) == 1%             if ((b19 or b18 or b17 or b16 or b15 or b14 or b13 or b12 or b11 or b10) = '1') then   -- check bit range [19  10]
        if bitorreduce(x, 20, 16) == 1%                 if ((b19 or b18 or b17 or b16 or b15) = '1') then   -- check bit range [19  15]
            if bitorreduce(x, 20, 18) == 1%                     if ((b19 or b18 or b17) = '1') then   -- check bit range [19  17]
                if bitorreduce(x, 20, 19) == 1%                         if ((b19 or b18) = '1') then   -- check bit range [19  18]
                    if bitorreduce(x, 20, 20) == 1%                             if (b19 = '1') then   -- [19]
                        lzc_count = fi(20,0,6,0);%                                 lzc_count <= "010100";  -- lzc = 20
                    else%                             else  -- check bit range [18]
                        lzc_count = fi(21,0,6,0);%                                 lzc_count <= "010101";  -- lzc = 21
                    end%                             end if;
                else%                         else  -- check bit range [17]
                    lzc_count = fi(22,0,6,0);%                             lzc_count <= "010110";  -- lzc = 22
                end%                         end if;
            else%                     else  -- check bit range [16  15]
                if bitorreduce(x, 17, 17) == 1%                         if (b16 = '1') then   -- [16]
                    lzc_count = fi(23,0,6,0);%                             lzc_count <= "010111";  -- lzc = 23
                else%                         else  -- check bit range [15]
                    lzc_count = fi(24,0,6,0);%                             lzc_count <= "011000";  -- lzc = 24
                end%                         end if;
            end%                     end if;
        else%                 else  -- check bit range [14  10]
            if bitorreduce(x, 15, 13) == 1%                     if ((b14 or b13 or b12) = '1') then   -- check bit range [14  12]
                if bitorreduce(x, 15, 14) == 1%                         if ((b14 or b13) = '1') then   -- check bit range [14  13]
                    if bitorreduce(x, 15, 15) == 1%                             if (b14 = '1') then   -- [14]
                        lzc_count = fi(25,0,6,0);%                                 lzc_count <= "011001";  -- lzc = 25
                    else%                             else  -- check bit range [13]
                        lzc_count = fi(26,0,6,0);%                                 lzc_count <= "011010";  -- lzc = 26
                    end%                             end if;
                else%                         else  -- check bit range [12]
                    lzc_count = fi(27,0,6,0);%                             lzc_count <= "011011";  -- lzc = 27
                end%                         end if;
            else%                     else  -- check bit range [11  10]
                if bitorreduce(x, 12, 12) == 1%                         if (b11 = '1') then   -- [11]
                    lzc_count = fi(28,0,6,0);%                             lzc_count <= "011100";  -- lzc = 28
                else%                         else  -- check bit range [10]
                    lzc_count = fi(29,0,6,0);%                             lzc_count <= "011101";  -- lzc = 29
                end%                         end if;
            end%                     end if;
        end%                 end if;
    else%             else  -- check bit range [9  0]
        if bitorreduce(x, 10, 6) == 1%                 if ((b9 or b8 or b7 or b6 or b5) = '1') then   -- check bit range [9  5]
            if bitorreduce(x, 10, 9) == 1%                     if ((b9 or b8 or b7) = '1') then   -- check bit range [9  7]
                if bitorreduce(x, 10, 9) == 1%                         if ((b9 or b8) = '1') then   -- check bit range [9  8]
                    if bitorreduce(x, 10, 10) == 1%                             if (b9 = '1') then   -- [9]
                        lzc_count = fi(30,0,6,0);%                                 lzc_count <= "011110";  -- lzc = 30
                    else%                             else  -- check bit range [8]
                        lzc_count = fi(31,0,6,0);%                                 lzc_count <= "011111";  -- lzc = 31
                    end%                             end if;
                else%                         else  -- check bit range [7]
                    lzc_count = fi(32,0,6,0);%                             lzc_count <= "100000";  -- lzc = 32
                end%                         end if;
            else%                     else  -- check bit range [6  5]
                if bitorreduce(x, 7, 7) == 1%                         if (b6 = '1') then   -- [6]
                    lzc_count = fi(33,0,6,0);%                             lzc_count <= "100001";  -- lzc = 33
                else%                         else  -- check bit range [5]
                    lzc_count = fi(34,0,6,0);%                             lzc_count <= "100010";  -- lzc = 34
                end%                         end if;
            end%                     end if;
        else%                 else  -- check bit range [4  0]
            if bitorreduce(x, 5, 3) == 1%                     if ((b4 or b3 or b2) = '1') then   -- check bit range [4  2]
                if bitorreduce(x, 5, 4) == 1%                         if ((b4 or b3) = '1') then   -- check bit range [4  3]
                    if bitorreduce(x, 5, 5) == 1%                             if (b4 = '1') then   -- [4]
                        lzc_count = fi(35,0,6,0);%                                 lzc_count <= "100011";  -- lzc = 35
                    else%                             else  -- check bit range [3]
                        lzc_count = fi(36,0,6,0);%                                 lzc_count <= "100100";  -- lzc = 36
                    end%                             end if;
                else%                         else  -- check bit range [2]
                    lzc_count = fi(37,0,6,0);%                             lzc_count <= "100101";  -- lzc = 37
                end%                         end if;
            else%                     else  -- check bit range [1  0]
                if bitorreduce(x, 2, 2) == 1%                         if (b1 = '1') then   -- [1]
                    lzc_count = fi(38,0,6,0);%                             lzc_count <= "100110";  -- lzc = 38
                else%                         else  -- check bit range [0]
                    lzc_count = fi(39,0,6,0);%                             lzc_count <= "100111";  -- lzc = 39
                end%                         end if;
            end%                     end if;
        end%                 end if;
    end%             end if;
end%         end if;
